simulink model "SystemeCompletProcedural_compared"  (R2019b)
settings: Solver=FixedStepAuto  StartTime=0.0  StopTime=5  FixedStep=0.0001  RelTol=1e-3
libraries: dspsrcs4 x2
settings Model: Creator=jeanz  LastModifiedBy=jeanz

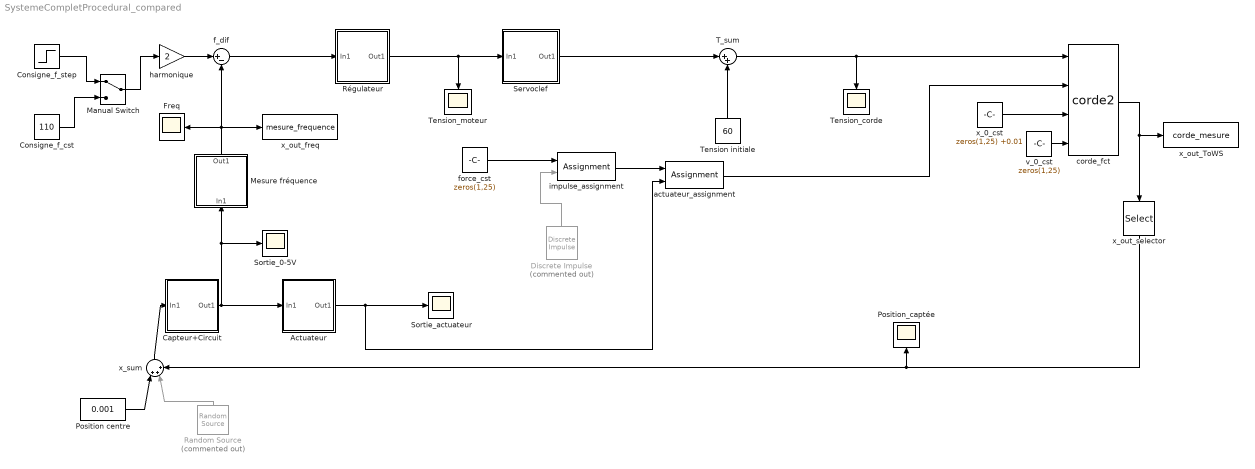
== system SystemeCompletProcedural_compared ==
  Actuateur : Subsystem
  Capteur+Circuit : Subsystem
  Consigne_f_cst : Constant  Value=110
  Consigne_f_step : Step  Time=3  Before=100  After=110  SampleTime=0
  Discrete Impulse : dspsrcs4/Discrete  Impulse  Commented=on  Delay=0  SampleTime=0.1  FrameSample=1  OutputFrames=off  dataType=double  isSigned=on  wordLen=16  udDataType=sfix(16)  fracBitsMode=Best precision  numFracBits=15  OutDataTypeStr=double  LastOutDataTypeStr=double
  Freq : Scope
  Manual Switch : ManualSwitch
  Mesure fréquence : Subsystem
  Position centre : Constant  Value=0.001
  Position_captée : Scope
  Random Source : dspsrcs4/Random Source  Commented=on  SrcType=Uniform  NormMethod=Ziggurat  CltLength=12  MinVal=-0.0001  MaxVal=0.0001  MeanVal=0  VarVal=1  RepMode=Not repeatable  rawSeed=1  IsInherit=off  SampMode=Discrete  SampTime=1  SampFrame=1  DataType=Double  OutComplex=Real  OutputFrames=off
  Régulateur : Subsystem
  Servoclef : Subsystem
  Sortie_0-5V : Scope
  Sortie_actuateur : Scope
  T_sum : Sum  Inputs=|++
  Tension initiale : Constant  Value=60
  Tension_corde : Scope
  Tension_moteur : Scope
  actuateur_assignment : Assignment  DiagnosticForDimensions=Warning  IndexOptions=Starting index (dialog)  Indices=20  OutputSizes=1
  corde_fct : M-S-Function  FunctionName=corde2  Parameters=0.00325, 0.44, 0.0326, 25
  f_dif : Sum  Inputs=|+-
  force_cst : Constant  Value=zeros(1,25)
  harmonique : Gain  Gain=2
  impulse_assignment : Assignment  DiagnosticForDimensions=Warning  IndexOptions=Starting index (dialog)  Indices=10  OutputSizes=1
  v_0_cst : Constant  Value=zeros(1,25)
  x_0_cst : Constant  Value=zeros(1,25) +0.01
  x_out_ToWS : ToWorkspace  VariableName=corde_mesure  SaveFormat=Timeseries  SampleTime=-1
      settings: Decimation=3
  x_out_freq : ToWorkspace  VariableName=mesure_frequence  SaveFormat=Timeseries  SampleTime=-1
      settings: Decimation=3
  x_out_selector : Selector  IndexOptions=Starting index (dialog)  Indices=6  OutputSizes=1
  x_sum : Sum  Inputs=|+++
  wires:
  corde_fct/1 -> x_out_selector/1, x_out_ToWS/1
  Actuateur/1(Out1) -> Sortie_actuateur/1, actuateur_assignment/2
  Capteur+Circuit/1(Out1) -> Mesure fréquence/1(In1), Sortie_0-5V/1, Actuateur/1(In1)
  Mesure fréquence/1(Out1) -> f_dif/2, Freq/1, x_out_freq/1
  x_sum/1 -> Capteur+Circuit/1(In1)
  x_out_selector/1 -> x_sum/3, Position_captée/1
  Position centre/1 -> x_sum/1
  T_sum/1 -> corde_fct/1, Tension_corde/1
  Random Source/1 -> x_sum/2
  Régulateur/1(Out1) -> Servoclef/1(In1), Tension_moteur/1
  f_dif/1 -> Régulateur/1(In1)
  actuateur_assignment/1 -> corde_fct/2
  Discrete Impulse/1 -> impulse_assignment/2
  impulse_assignment/1 -> actuateur_assignment/1
  force_cst/1 -> impulse_assignment/1
  x_0_cst/1 -> corde_fct/3
  v_0_cst/1 -> corde_fct/4
  harmonique/1 -> f_dif/1
  Consigne_f_step/1 -> Manual Switch/1
  Manual Switch/1 -> harmonique/1
  Consigne_f_cst/1 -> Manual Switch/2
  Servoclef/1(Out1) -> T_sum/1
  Tension initiale/1 -> T_sum/2

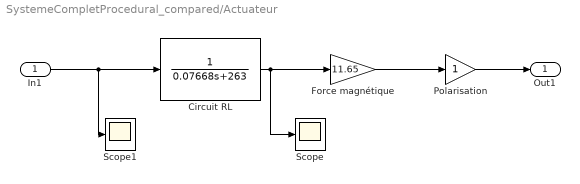
== system SystemeCompletProcedural_compared/Actuateur ==
  In1 : Inport
  Circuit RL : TransferFcn  Denominator=[0.07668 263]
  Force magnétique : Gain  Gain=11.65
  Polarisation : Gain
  Scope : Scope
  Scope1 : Scope
  Out1 : Outport
  wires:
  Circuit RL/1 -> Force magnétique/1, Scope/1
  In1/1 -> Scope1/1, Circuit RL/1
  Force magnétique/1 -> Polarisation/1
  Polarisation/1 -> Out1/1

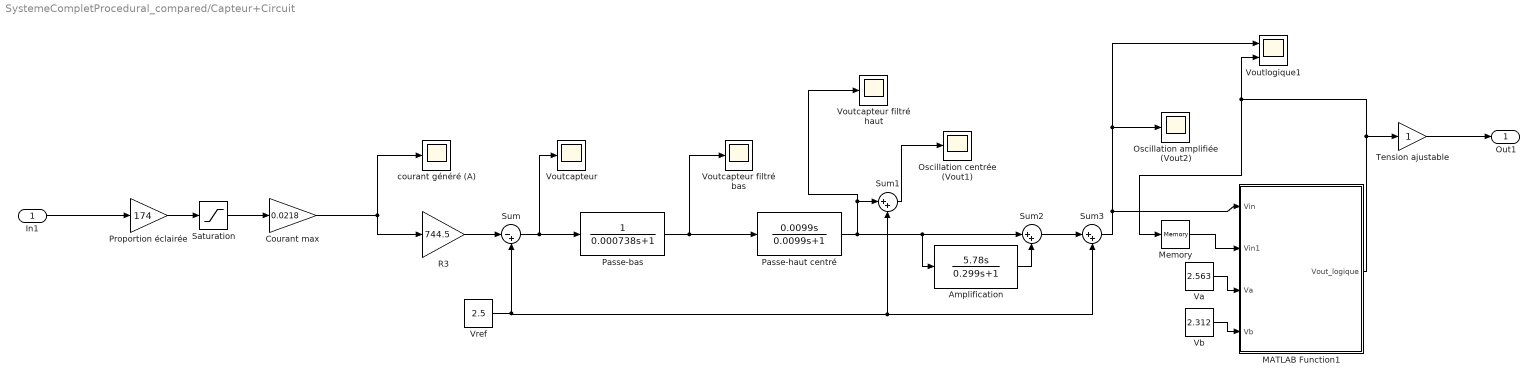
== system SystemeCompletProcedural_compared/Capteur+Circuit ==
  In1 : Inport
  "Amplification " : TransferFcn  Numerator=[5.78 0]  Denominator=[0.299 1]
  Courant max : Gain  Gain=0.0218
  MATLAB Function1 : MATLAB Function  TreatAsAtomicUnit=on
  Memory : Memory
  "Oscillation amplifiée (Vout2) " : Scope
  Oscillation centrée (Vout1) : Scope
  Passe-bas : TransferFcn  Denominator=[0.000738 1]
  "Passe-haut centré " : TransferFcn  Numerator=[0.0099 0]  Denominator=[0.0099 1]
  Proportion éclairée : Gain  Gain=174
  R3 : Gain  Gain=744.5
  Saturation : Saturate  UpperLimit=0.497  LowerLimit=0
  Sum : Sum  Inputs=|-+
  Sum1 : Sum  Inputs=|++
  Sum2 : Sum  Inputs=|++
  Sum3 : Sum  Inputs=|++
  Tension ajustable : Gain
  "Va " : Constant  Value=2.563
  Vb : Constant  Value=2.312
  "Voutcapteur " : Scope
  Voutcapteur filtré bas : Scope
  Voutcapteur filtré haut : Scope
  Voutlogique1 : Scope  NumInputPorts=2
  "Vref " : Constant  Value=2.5
  "courant généré (A) " : Scope
  Out1 : Outport
  wires:
  "Amplification "/1 -> Sum2/2
  Sum3/1 -> Voutlogique1/1, "Oscillation amplifiée (Vout2) "/1, MATLAB Function1/1(Vin)
  "Vref "/1 -> Sum/2, Sum3/2, Sum1/2
  Sum/1 -> "Voutcapteur "/1, Passe-bas/1
  R3/1 -> Sum/1
  "Passe-haut centré "/1 -> Sum2/1, "Amplification "/1, Voutcapteur filtré haut/1, Sum1/1
  Vb/1 -> MATLAB Function1/4(Vb)
  Passe-bas/1 -> Voutcapteur filtré bas/1, "Passe-haut centré "/1
  Sum2/1 -> Sum3/1
  Sum1/1 -> Oscillation centrée (Vout1)/1
  MATLAB Function1/1(Vout_logique) -> Memory/1, Voutlogique1/2, Tension ajustable/1
  "Va "/1 -> MATLAB Function1/3(Va)
  Saturation/1 -> Courant max/1
  Proportion éclairée/1 -> Saturation/1
  Courant max/1 -> R3/1, "courant généré (A) "/1
  In1/1 -> Proportion éclairée/1
  Memory/1 -> MATLAB Function1/2(Vin1)
  Tension ajustable/1 -> Out1/1

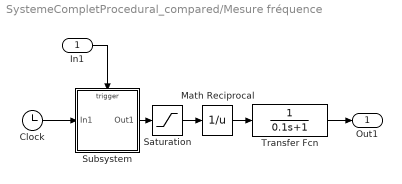
== system SystemeCompletProcedural_compared/Mesure fréquence ==
  In1 : Inport
  Clock : Clock
  Math Reciprocal : Math  Operator=reciprocal  SaturateOnIntegerOverflow=on
  Saturation : Saturate  UpperLimit=1  LowerLimit=0.003
  Subsystem : Subsystem
  Transfer Fcn : TransferFcn  Denominator=[0.1 1]
  Out1 : Outport
  wires:
  In1/1 -> Subsystem/Trigger
  Clock/1 -> Subsystem/1(In1)
  Subsystem/1(Out1) -> Saturation/1
  Saturation/1 -> Math Reciprocal/1
  Math Reciprocal/1 -> Transfer Fcn/1
  Transfer Fcn/1 -> Out1/1

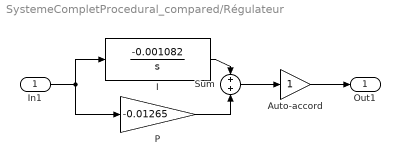
== system SystemeCompletProcedural_compared/Régulateur ==
  In1 : Inport
  Auto-accord : Gain
  I : TransferFcn  Numerator=[-0.001082]  Denominator=[1 0]
  P : Gain  Gain=-0.01265
  Sum : Sum  Inputs=+|+
  Out1 : Outport
  wires:
  In1/1 -> P/1, I/1
  I/1 -> Sum/1
  P/1 -> Sum/2
  Sum/1 -> Auto-accord/1
  Auto-accord/1 -> Out1/1

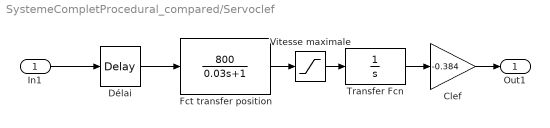
== system SystemeCompletProcedural_compared/Servoclef ==
  In1 : Inport
  Clef : Gain  Gain=-0.384
  Délai : TransportDelay  DelayTime=0.01
  Fct transfer position : TransferFcn  Numerator=[800]  Denominator=[0.03 1]
  Transfer Fcn : TransferFcn  Denominator=[1 0]
  Vitesse maximale : Saturate  UpperLimit=1000  LowerLimit=-1000
  Out1 : Outport
  wires:
  Délai/1 -> Fct transfer position/1
  In1/1 -> Délai/1
  Clef/1 -> Out1/1
  Fct transfer position/1 -> Vitesse maximale/1
  Transfer Fcn/1 -> Clef/1
  Vitesse maximale/1 -> Transfer Fcn/1

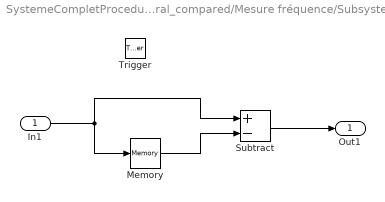
== system SystemeCompletProcedural_compared/Mesure fréquence/Subsystem ==
  In1 : Inport
  Trigger : TriggerPort  VariantControl=Variant  PortDimensions=1
  Memory : Memory  InheritSampleTime=on
  Subtract : Sum  Inputs=+-
  Out1 : Outport
  wires:
  Memory/1 -> Subtract/2
  Subtract/1 -> Out1/1
  In1/1 -> Memory/1, Subtract/1

== matlab function SystemeCompletProcedural_compared/Capteur+Circuit/MATLAB Function1 ==
  data: Vin input; Vin1 input; Vout_logique output; Va input; Vb input
function Vout_logique = fcn(Vin, Vin1 , Va, Vb)
Vout_logique = Vin1;
if Vin > Va && Vin1 == 5
    Vout_logique = 0;
end
if Vin < Vb && Vin1 == 0
    Vout_logique = 5;
end
end
